simulink model "Q6_Model"  (R2025b)
settings: Solver=VariableStepAuto  StartTime=0.0  StopTime=10.0  RelTol=1e-3
values from neighbouring files (symbols this model uses):
  D = [0 0]'    [main.m]
  I_5 = eye(5)    [main.m]
  K = lqr(A, B, Qr, Rr)    [IP_MACRO.m]
  x0 = [0.1 0 0 0 0]'    [main.m]
undefined symbols (not defined in the file or in its folder): A, B
settings Model: Creator=lucas  LastModifiedBy=texman

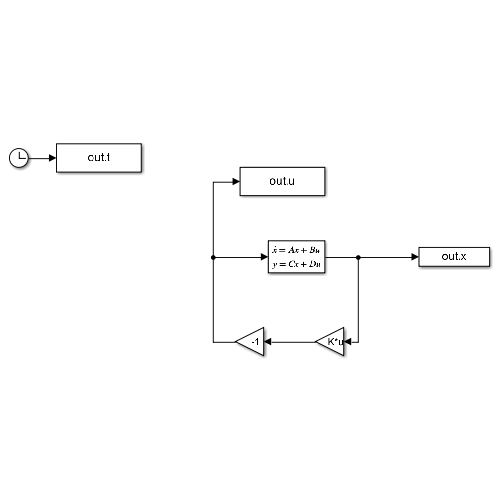
[thumbnail: Simulink's stored preview of the top-level diagram]
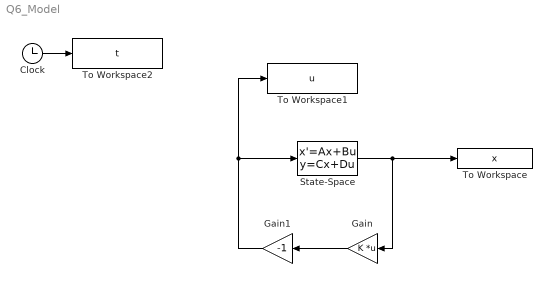
== system Q6_Model ==
  Clock : Clock
  Gain : Gain  Gain=K  Multiplication=Matrix(K*u)
  Gain1 : Gain  Gain=-1
  State-Space : StateSpace  A=A  B=B  C=I_5  D=D  InitialCondition=x0  ContinuousStateAttributes={'x1','x2','x3','x4','x5'}
  To Workspace : ToWorkspace  VariableName=x  SaveFormat=Timeseries  SampleTime=-1
  To Workspace1 : ToWorkspace  VariableName=u  SaveFormat=Timeseries  SampleTime=-1
  To Workspace2 : ToWorkspace  VariableName=t  SaveFormat=Timeseries  SampleTime=-1
  wires:
  State-Space/1 -> To Workspace/1, Gain/1
  Gain/1 -> Gain1/1
  Gain1/1 -> To Workspace1/1, State-Space/1
  Clock/1 -> To Workspace2/1
